simulink model "controller_test_module"  (R2024b)
settings: Solver=ode4  StartTime=0.0  StopTime=1  FixedStep=1e-5  RelTol=1e-3
libraries: dspsrcs4 x1
settings Model: Creator=javnson  LastModifiedBy=javnson

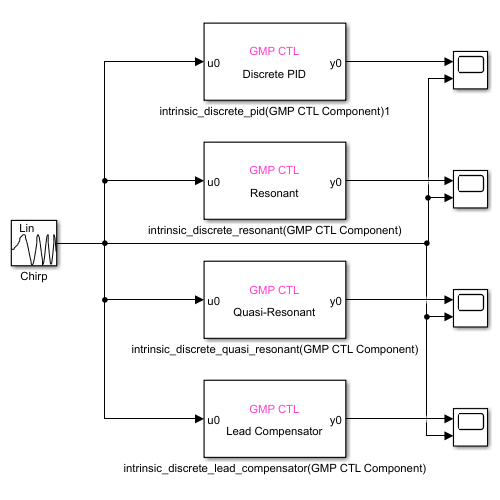
[thumbnail: Simulink's stored preview of the top-level diagram]
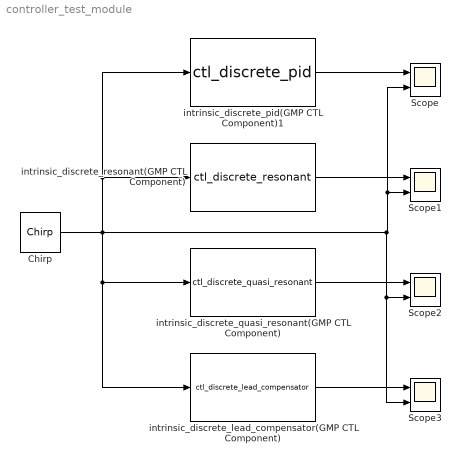
== system controller_test_module ==
  Chirp : dspsrcs4/Chirp  sweep=Linear  mode=Unidirectional  f0=100  f1=1000  t1=1  Tsweep=1  phase=0  Ts=1e-5  spf=1  datatype=double  OutputFrames=off
  Scope{,1..3} (4 alike) : Scope  NumInputPorts=2
  intrinsic_discrete_lead_compensator(GMP CTL Component) : S-Function  FunctionName=ctl_discrete_lead_compensator  Parameters=[1.0; 0.707],1/1e-5  SFunctionModules=ctl_discrete_lead_compensator_wrapper.cpp ctl_component_discrete ctl_component_basic ctl_component_continuous ctl_component_protection ctl_component_advance  SFunctionDeploymentMode=off  EnableBusSupport=off  mask(S-Function Builder){}
      mask help: Simulink:masks:SFunctionBuilder_MD
      mask init:
      | val = [[.9  0.75 0.75 1 1 .9 .9 1]',[1 1 0.75 0.75 .9 .9 1 .9]'];try , sys = get_param(gcb,'SfunBuilderFcnName');if isempty(sys), sys = get_param(gcb,'FunctionName'); end,catch, sys = get_param(gcb,'FunctionName'); end
      settings: CopyFcn=set_param(gcbh,'LinkStatus','none')  OpenFcn=sfunctionwizard(gcbh)
      mask Display:
      | %plot(val(:,1),val(:,2))
      | %disp(sys)
      | port_label('input',1,sprintf('%s', 'u0'),'interpreter','tex')
      | port_label('output',1,sprintf('%s', 'y0'),'interpreter','tex')
      | 
      | color('magenta');
      | text(0.5, 0.65, 'GMP CTL', 'horizontalAlignment', 'center');
      | 
      | color('black');
      | text(0.5, 0.35, 'Lead Compensator', 'horizontalAlignment', 'center');
  intrinsic_discrete_pid(GMP CTL Component)1 : S-Function  FunctionName=ctl_discrete_pid  Parameters=[0.5; 0.0001; 0.0001],[-10,10],1/1e-5  SFunctionModules=ctl_discrete_pid_wrapper.cpp ctl_component_discrete ctl_component_basic ctl_component_continuous ctl_component_protection ctl_component_advance  SFunctionDeploymentMode=off  EnableBusSupport=off  mask(S-Function Builder){}
      mask help: Simulink:masks:SFunctionBuilder_MD
      mask init: same as controller_test_module/intrinsic_discrete_lead_compensator(GMP CTL Component)
      settings: CopyFcn=set_param(gcbh,'LinkStatus','none')  OpenFcn=sfunctionwizard(gcbh)
      mask Display:
      | %plot(val(:,1),val(:,2))
      | %disp(sys)
      | port_label('input',1,sprintf('%s', 'u0'),'interpreter','tex')
      | port_label('output',1,sprintf('%s', 'y0'),'interpreter','tex')
      | 
      | color('magenta');
      | text(0.5, 0.65, 'GMP CTL', 'horizontalAlignment', 'center');
      | 
      | color('black');
      | text(0.5, 0.35, 'Discrete PID', 'horizontalAlignment', 'center');
  intrinsic_discrete_quasi_resonant(GMP CTL Component) : S-Function  FunctionName=ctl_discrete_quasi_resonant  Parameters=[0.5; 350.0; 0.5],1/1e-5  SFunctionModules=ctl_discrete_quasi_resonant_wrapper.cpp ctl_component_discrete ctl_component_basic ctl_component_continuous ctl_component_protection ctl_component_advance  SFunctionDeploymentMode=off  EnableBusSupport=off  mask(S-Function Builder){}
      mask help: Simulink:masks:SFunctionBuilder_MD
      mask init: same as controller_test_module/intrinsic_discrete_lead_compensator(GMP CTL Component)
      settings: CopyFcn=set_param(gcbh,'LinkStatus','none')  OpenFcn=sfunctionwizard(gcbh)
      mask Display:
      | port_label('input',1,sprintf('%s', 'u0'),'interpreter','tex')
      | port_label('output',1,sprintf('%s', 'y0'),'interpreter','tex')
      | 
      | color('magenta');
      | text(0.5, 0.65, 'GMP CTL', 'horizontalAlignment', 'center');
      | 
      | color('black');
      | text(0.5, 0.35, 'Quasi-Resonant', 'horizontalAlignment', 'center');
  intrinsic_discrete_resonant(GMP CTL Component) : S-Function  FunctionName=ctl_discrete_resonant  Parameters=[0.5; 350.0],1/1e-5  SFunctionModules=ctl_discrete_resonant_wrapper.cpp ctl_component_discrete ctl_component_basic ctl_component_continuous ctl_component_protection ctl_component_advance  SFunctionDeploymentMode=off  EnableBusSupport=off  mask(S-Function Builder){}
      mask help: Simulink:masks:SFunctionBuilder_MD
      mask init: same as controller_test_module/intrinsic_discrete_lead_compensator(GMP CTL Component)
      settings: CopyFcn=set_param(gcbh,'LinkStatus','none')  OpenFcn=sfunctionwizard(gcbh)
      mask Display:
      | port_label('input',1,sprintf('%s', 'u0'),'interpreter','tex')
      | port_label('output',1,sprintf('%s', 'y0'),'interpreter','tex')
      | 
      | color('magenta');
      | text(0.5, 0.65, 'GMP CTL', 'horizontalAlignment', 'center');
      | 
      | color('black');
      | text(0.5, 0.35, 'Resonant', 'horizontalAlignment', 'center');
  wires:
  Chirp/1 -> Scope3/2, Scope2/2, Scope/2, Scope1/2, intrinsic_discrete_lead_compensator(GMP CTL Component)/1, intrinsic_discrete_quasi_resonant(GMP CTL Component)/1, intrinsic_discrete_resonant(GMP CTL Component)/1, intrinsic_discrete_pid(GMP CTL Component)1/1
  intrinsic_discrete_pid(GMP CTL Component)1/1 -> Scope/1
  intrinsic_discrete_resonant(GMP CTL Component)/1 -> Scope1/1
  intrinsic_discrete_quasi_resonant(GMP CTL Component)/1 -> Scope2/1
  intrinsic_discrete_lead_compensator(GMP CTL Component)/1 -> Scope3/1
